simulink model "closed_observer"  (R2024a)
settings: Solver=VariableStepAuto  StartTime=0.0  StopTime=10  MaxStep=1e-3  RelTol=1e-3
values from neighbouring files (symbols this model uses):
  A = [0 1; -3 4]    [init2.m]
  Ab = [G,          zeros(n_w, n) ... (first row only)    [init2.m]
  B = [3 -5; 2 0]    [init2.m]
  Bb = [zeros(n_w, size(B, 2)) ... (first row only)    [init2.m]
  Bf = [3 1; 2 0]    [init2.m]
  C = [4 1; -2 0]    [init2.m]
  Ct = [Cb ... (first row only)    [init2.m]
  Cz = [3 1; 2 0]    [init2.m]
  D = [2 0; 0 -3]    [init2.m]
  Df = [-1 0; 0 1]    [init2.m]
  Dt = [D ... (first row only)    [init2.m]
  Dz = [-2 0; 0 1]    [init2.m]
  G = [0 2 0 0 0 0 ... (first row only)    [init2.m]
  K = -Y * inv(P)    [init2.m]
  Kw = Dz_inv * (Yg - F*P)    [init2.m]
  L = place(Ab', Ct', lambda_obs)'    [init2.m]
  w0 = [1 0 1 0 1 0]'    [init2.m]
  x0 = [1; 1]    [init2.m]
  xe0 = [0 0 0 0 0 0 0 0]'    [init2.m]
  Y1 = [0 -5 0 0 0 0; 0 0 5 0 0 0]    [init2.m]
  Y2 = [0 0 3 0 0 0; 0 -1 0 0 0 0]    [init2.m]
  Yg = [0 0 0 0 4 0; 0 0 0 0 0 -3]    [init2.m]
settings Model: NumberOfSteps=2  Creator=eva  LastModifiedBy=eva

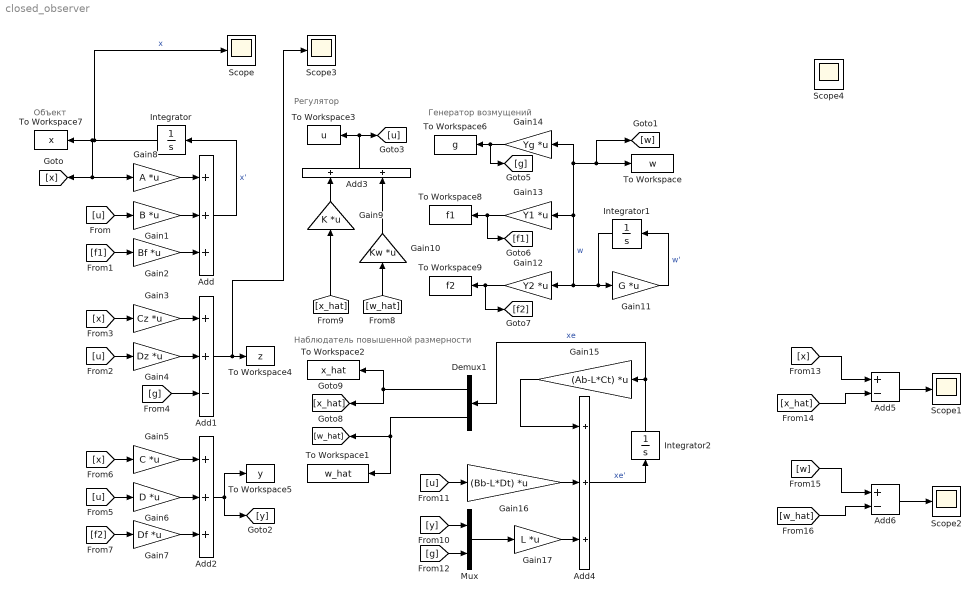
== system closed_observer ==
  note: Наблюдатель повышенной размерности
  note: Генератор возмущений
  note: Регулятор
  note: Объект
  Add : Sum  Inputs=+++
  Add1 : Sum  Inputs=++-
  Add2 : Sum  Inputs=+++
  Add3 : Sum
  Add4 : Sum  Inputs=+++
  Add5 : Sum  Inputs=+-
  Add6 : Sum  Inputs=+-
  Demux1 : Demux  Outputs=[2,6]
  Gain1 : Gain  Gain=B  Multiplication=Matrix(K*u)
  Gain10 : Gain  Gain=Kw  Multiplication=Matrix(K*u)
  Gain11 : Gain  Gain=G  Multiplication=Matrix(K*u)
  Gain12 : Gain  Gain=Y2  Multiplication=Matrix(K*u)
  Gain13 : Gain  Gain=Y1  Multiplication=Matrix(K*u)
  Gain14 : Gain  Gain=Yg  Multiplication=Matrix(K*u)
  Gain15 : Gain  Gain=(Ab-L*Ct)  Multiplication=Matrix(K*u)
  Gain16 : Gain  Gain=(Bb-L*Dt)  Multiplication=Matrix(K*u)
  Gain17 : Gain  Gain=L  Multiplication=Matrix(K*u)
  Gain2 : Gain  Gain=Bf  Multiplication=Matrix(K*u)
  Gain3 : Gain  Gain=Cz  Multiplication=Matrix(K*u)
  Gain4 : Gain  Gain=Dz  Multiplication=Matrix(K*u)
  Gain5 : Gain  Gain=C  Multiplication=Matrix(K*u)
  Gain6 : Gain  Gain=D  Multiplication=Matrix(K*u)
  Gain7 : Gain  Gain=Df  Multiplication=Matrix(K*u)
  Gain8 : Gain  Gain=A  Multiplication=Matrix(K*u)
  Gain9 : Gain  Gain=K  Multiplication=Matrix(K*u)
  Integrator : Integrator  InitialCondition=x0
  Integrator1 : Integrator  InitialCondition=w0
  Integrator2 : Integrator  InitialCondition=xe0
  Mux : Mux  Inputs=2
  Scope{,1..4} (5 alike) : Scope
  To Workspace : ToWorkspace  VariableName=w  SaveFormat=Timeseries  SampleTime=-1
  To Workspace1 : ToWorkspace  VariableName=w_hat  SaveFormat=Timeseries  SampleTime=-1
  To Workspace2 : ToWorkspace  VariableName=x_hat  SaveFormat=Timeseries  SampleTime=-1
  To Workspace3 : ToWorkspace  VariableName=u  SaveFormat=Timeseries  SampleTime=-1
  To Workspace4 : ToWorkspace  VariableName=z  SaveFormat=Timeseries  SampleTime=-1
  To Workspace5 : ToWorkspace  VariableName=y  SaveFormat=Timeseries  SampleTime=-1
  To Workspace6 : ToWorkspace  VariableName=g  SaveFormat=Timeseries  SampleTime=-1
  To Workspace7 : ToWorkspace  VariableName=x  SaveFormat=Timeseries  SampleTime=-1
  To Workspace8 : ToWorkspace  VariableName=f1  SaveFormat=Timeseries  SampleTime=-1
  To Workspace9 : ToWorkspace  VariableName=f2  SaveFormat=Timeseries  SampleTime=-1
  wires:
  Gain8/1 -> Add/1
  Gain1/1 -> Add/2
  Gain2/1 -> Add/3
  Add/1 -> Integrator/1  "x'"
  Integrator/1 -> Scope/1, To Workspace7/1, Gain8/1, [x]  "x"
  [u] -> Gain1/1
  [f1] -> Gain2/1
  [u] -> Gain4/1
  [x] -> Gain3/1
  Gain3/1 -> Add1/1
  Gain4/1 -> Add1/2
  [g] -> Add1/3
  Add1/1 -> Scope3/1, To Workspace4/1
  Add2/1 -> To Workspace5/1, [y]
  Gain6/1 -> Add2/2
  Gain5/1 -> Add2/1
  [x] -> Gain5/1
  [u] -> Gain6/1
  Gain7/1 -> Add2/3
  [f2] -> Gain7/1
  [w_hat] -> Gain10/1
  [x_hat] -> Gain9/1
  Gain9/1 -> Add3/1
  Gain10/1 -> Add3/2
  Add3/1 -> To Workspace3/1, [u]
  Gain11/1 -> Integrator1/1  "w'"
  Integrator1/1 -> Gain11/1, Gain14/1, [w], To Workspace/1, Gain13/1, Gain12/1  "w"
  Gain14/1 -> [g], To Workspace6/1
  Gain13/1 -> [f1], To Workspace8/1
  Gain12/1 -> To Workspace9/1, [f2]
  Mux/1 -> Gain17/1
  [u] -> Gain16/1
  Gain16/1 -> Add4/2
  Gain17/1 -> Add4/3
  Gain15/1 -> Add4/1
  Add4/1 -> Integrator2/1  "xe'"
  Integrator2/1 -> Demux1/1, Gain15/1  "xe"
  [y] -> Mux/1
  [g] -> Mux/2
  Demux1/1 -> [x_hat], To Workspace2/1
  Demux1/2 -> To Workspace1/1, [w_hat]
  [x] -> Add5/1
  [x_hat] -> Add5/2
  Add5/1 -> Scope1/1
  Add6/1 -> Scope2/1
  [w_hat] -> Add6/2
  [w] -> Add6/1
